simulink model "H2DFRL_LExCI_env_2018a"  (R2018a)
settings: Solver=FixedStepAuto  StartTime=0.0  StopTime=50  FixedStep=0.08  RelTol=1e-3
values from neighbouring files (symbols this model uses):
  action_mean_selector_ppo = 1:num_actions    [ReinforcementLearningBlockInit_H2DFRL.m]
  action_sampling_mode = 1    [ReinforcementLearningBlockInit_H2DFRL.m]
  action_selector_ddpg = 1:num_actions    [ReinforcementLearningBlockInit_H2DFRL.m]
  action_std_selector_ppo = 1:num_actions    [ReinforcementLearningBlockInit_H2DFRL.m]
  action_type = 1    [ReinforcementLearningBlockInit_H2DFRL.m]
  C2C_NMPC = init_C2C_NMPC_H2DF(C2C_NMPC.expdata)    [init_H2DFRL_GRU.m]
  num_actions = 4    [ReinforcementLearningBlockInit_H2DFRL.m]
  rl_algorithm = 1    [ReinforcementLearningBlockInit_H2DFRL.m]
undefined symbols (not defined in the file or in its folder): CA50_offset, DiscIntNeverNeededParam, enable_CA50_noise, enable_CA50_offset, enable_IMEP_noise, enable_IMEP_offset, IMEP_offset, NUMBER_OF_ACTIONS
libraries: simulink x15, dspsrcs4 x4
(part 2 of 3)

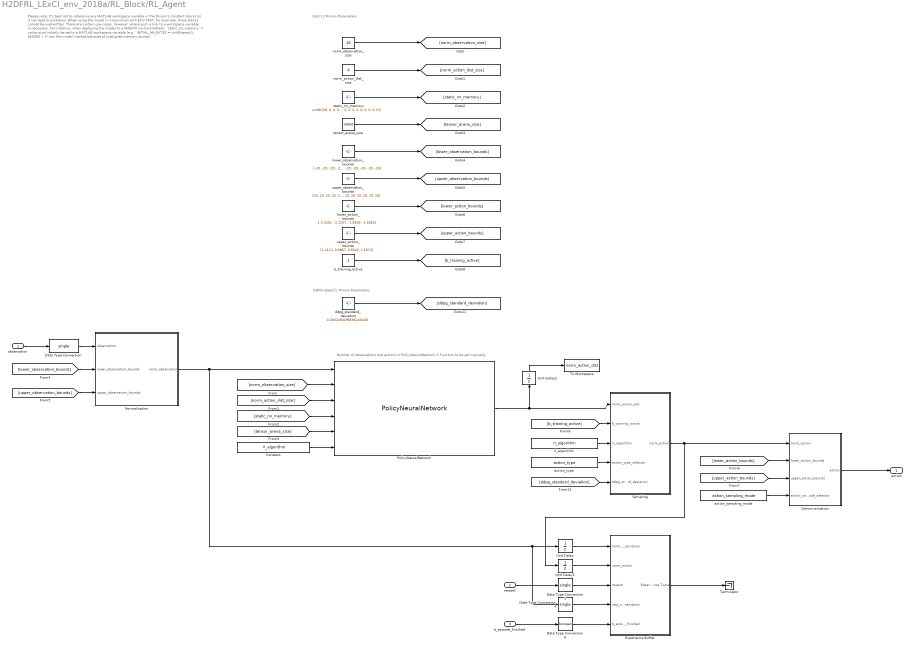
== system H2DFRL_LExCI_env_2018a/RL_Block/RL_Agent ==
  note: LExCI 2 Minion Parameters
  note: DDPG-Specific Minion Parameters
  note: Number of observations and actions in PolicyNeuralNetwork S-Function to be set manually.
  note: Please note:
      |
      | It's best not to reference any MATLAB workspace variable in the Minion's constant blocks as it can lead to
      | problems. When using the model in conjunction with ECU-TEST, for example, those blocks cannot be
      | overwritten.
      |
      | There are certain use-cases, however, where such a link to a workspace variable is necessary. For
      | instance, when deploying the model to a MABXIII via ControlDesk, `static_nn_memory`'s value must
      | initially be set to a MATLAB workspace variable (e.g. `INITIAL_NN_BYTES = uint8(zeros(1, 65536))`). If
      | not, the model crashes because of unaligned memory access.
  observation : Inport
  reward : Inport  Port=2
  b_episode_finished : Inport  Port=3
  Constant : Constant  Value=rl_algorithm  OutDataTypeStr=uint32
  Data Type Conversion : DataTypeConversion  OutDataTypeStr=single
  Data Type Conversion3 : DataTypeConversion  OutDataTypeStr=single
  Data Type Conversion4 : DataTypeConversion  OutDataTypeStr=single
  Data Type Conversion6 : DataTypeConversion  OutDataTypeStr=boolean
  Denormalization : Subsystem
  Experience Buffer : Subsystem
  Normalization : Subsystem
  PolicyNeuralNetwork : S-Function  InitFcn=try, set_param(gcb,'FunctionName','PolicyNeuralNetwork'), end  FunctionName=PolicyNeuralNetwork  SFunctionModules=PolicyNeuralNetwork_wrapper.cpp activations activations_common add add_common add_n arg_min_max assign_variable batch_to_space_nd broadcast_args broadcast_to call_once cast ceil circular_buffer circular_buffer_common comparisons concatenation conv conv_common cumsum depth_to_space depthwise_conv depthwise_conv_common dequantize dequantize_common detection_postprocess div elementwise elu ethosu exp expand_dims fill floor floor_div floor_mod fully_connected fully_connected_common gather gather_nd hard_swish hard_swish_common if kernel_runner kernel_util_micro l2norm l2_pool_2d leaky_relu leaky_relu_common logical logical_common logistic logistic_common log_softmax lstm_eval maximum_minimum micro_tensor_utils mirror_pad mul mul_common neg pack pad pooling pooling_common prelu prelu_common quantize quantize_common read_variable reduce reduce_common reshape resize_bilinear resize_nearest_neighbor round shape slice softmax softmax_common space_to_batch_nd space_to_depth split split_v squared_difference squeeze strided_slice sub sub_common svdf svdf_common tanh transpose transpose_conv unidirectional_sequence_lstm unpack var_handle while zeros_like flatbuffer_conversions op_resolver tensor_utils error_reporter schema_utils kernel_util portable_tensor_utils quantization_util common memory_helpers all_ops_resolver micro_graph micro_error_reporter micro_context micro_profiler test_helpers recording_micro_allocator micro_interpreter micro_time micro_resource_variable test_helper_custom_ops flatbuffer_utils mock_micro_graph debug_log micro_allocation_info system_setup micro_allocator micro_string micro_utils fake_micro_context persistent_arena_buffer_allocator recording_single_arena_buffer_allocator non_persistent_arena_buffer_allocator single_arena_buffer_allocator greedy_memory_planner linear_memory_planner non_persistent_buffer_planner_shim  SFunctionDeploymentMode=off  EnableBusSupport=off  mask(S-Function Builder){}
      mask help: Simulink:masks:SFunctionBuilder_MD
      mask init:
      | val = [[.9  0.75 0.75 1 1 .9 .9 1]',[1 1 0.75 0.75 .9 .9 1 .9]'];try , sys = get_param(gcb,'SfunBuilderFcnName');if isempty(sys), sys = get_param(gcb,'FunctionName'); end,catch, sys = get_param(gcb,'FunctionName'); end
      settings: CopyFcn=set_param(gcbh,'LinkStatus','none')  PreSaveFcn=try, set_param(gcb,'FunctionName','PolicyNeuralNetwork'), end  OpenFcn=sfunctionwizard(gcbh)
      mask Display: plot(val(:,1),val(:,2)),disp(sys),port_label('input',1,'norm_observation'),port_label('input',2,'norm_observation_size'),port_label('input',3,'norm_action_dist_size'),port_label('input',4,'static_nn_memory'),port_label('input',5,'tensor_arena_size'),port_label('input',6,'rl_algorithm'),port_label('output',1,'norm_action_dist')
  Sampling : Subsystem
  Terminator : Terminator
  To Workspace : ToWorkspace  VariableName=norm_action_dist  SampleTime=-1
  Unit Delay : UnitDelay  InitialCondition=-1*ones(16,1)  SampleTime=-1  HasFrameUpgradeWarning=on
  Unit Delay1 : UnitDelay  InitialCondition=-1*ones(4,1)  SampleTime=-1  HasFrameUpgradeWarning=on
  Unit Delay2 : UnitDelay  InitialCondition=-1*ones(4,1)  SampleTime=-1  HasFrameUpgradeWarning=on
  action_sampling_mode : Constant  Value=action_sampling_mode  OutDataTypeStr=uint8
  action_type : Constant  Value=action_type  OutDataTypeStr=uint8
  b_training_active : Constant  OutDataTypeStr=boolean
  ddpg_standard_deviation : Constant  Value=0.0002450298596240448  OutDataTypeStr=single
  lower_action_bounds : Constant  Value=[-2.3201, -2.1257, -1.8309, -1.6562]  OutDataTypeStr=single
  lower_observation_bounds : Constant  Value=[-20, -20, -20, -20, -20, -20, -20, -20, -20, -20, -20, -20, -20, -20, -20, -20]  OutDataTypeStr=single
  norm_action_dist_size : Constant  Value=4  OutDataTypeStr=uint32
  norm_observation_size : Constant  Value=16  OutDataTypeStr=uint32
  rl_algorithm : Constant  Value=rl_algorithm  OutDataTypeStr=uint8
  static_nn_memory : Constant  Value=uint8([28, 0, 0, 0, 84, 70, 76, 51, 0, 0, 18, 0, 28, 0, 24, 0, 20, 0, 16, 0, 12, 0, 8, 0, 0, 0, 4, 0, 18, 0, 0, 0, 24, 0, 0, 0, 104, 0, 0, 0, 140, 87, 0, 0, 156, 87, 0, 0, 228, 91, 0, 0, 3, 0, 0, 0, 2, 0, 0, 0, 44, 0, 0, 0, 4, 0, 0, 0, 40, 167, 255, 255, 12, 0, 0, 0, 4, 0, 0, 0, 19, 0, 0, 0, 67, 79, 78, 86, 69, 82, 83, 73, 79, 78, 95, 77, 69, 84, 65, 68, 65, 84, 65, 0, 76, 167, 255, 255, 11, 0, 0, 0, 4, 0, 0, 0, 19, 0, 0, 0, 109, 105, 110, 95, 114, 117, 110, 116, 105, 109, 101, 95, 118, 101, 114, 115, 105, 111, 110, 0, 13, 0, 0, 0, 32, 87, 0, 0, 0, 87, 0, 0, 232, 82, 0, 0, 216, 81, 0, 0, 200, 17, 0, 0, 184, 16, 0, 0, 168, 0, 0, 0, 160, 0, 0, 0, 152, 0, 0, 0, 144, 0, 0, 0, 136, 0, 0, 0, 104, 0, 0, 0, 4, 0, 0, 0, 54, 169, 255, 255, 4, 0, 0, 0, 84, 0, 0, 0, 12, 0, 0, 0, 8, 0, 14, 0, 8, 0, 4, 0, 8, 0, 0, 0, 16, 0, 0, 0, 36, 0, 0, 0, 0, 0, 6, 0, 8, 0, 4, 0, 6, 0, 0, 0, 4, 0, 0, 0, 0, 0, 0, 0, 0, 0, 10, 0, 16, 0, 12, 0, 8, 0, 4, 0, 10, 0, 0, 0, 2, 0, 0, 0, 2, 0, 0, 0, 4, 0, 0, 0, 6, 0, 0, 0, 50, 46, 49, 49, 46, 48, 0, 0, 150, 169, 255, 255, 4, 0, 0, 0, 16, 0, 0, 0, 49, 46, 53, 46, 48, 0, 0, 0, 0, 0, 0, 0, 0, 0, 0, 0, 80, 165, 255, 255, 84, 165, 255, 255, 88, 165, 255, 255, 92, 165, 255, 255, 194, 169, 255, 255, 4, 0, 0, 0, 0, 16, 0, 0, 195, 223, 248, 189, 165, 31, 134, 190, 238, 188, 71, 190, 121, 25, 100, 61, 240, 30, 182, 62, 66, 76, 196, 62, 202, 153, 72, 62, 139, 246, 211, 62, 185, 186, 23, 62, 196, 184, 59, 187, 236, 226, 53, 62, 128, 12, 9, 62, 67, 184, 120, 190, 173, 251, 162, 61, 146, 161, 55, 62, 148, 61, 179, 61, 220, 26, 78, 190, 129, 180, 236, 189, 201, 75, 95, 190, 158, 183, 249, 189, 54, 96, 9, 63, 14, 146, 237, 62, 146, 198, 19, 62, 129, 196, 40, 63, 237, 95, 204, 61, 193, 152, 236, 61, 42, 40, 87, 61, 27, 65, 222, 61, 75, 187, 23, 190, 145, 60, 6, 62, 176, 168, 115, 61, 9, 169, 14, 62, 178, 221, 16, 61, 40, 251, 84, 61, 173, 58, 218, 189, 173, 130, 55, 62, 66, 127, 175, 189, 163, 58, 143, 59, 62, 42, 119, 61, 238, 82, 2, 62, 197, 39, 121, 62, 149, 60, 136, 189, 43, 33, 133, 62, 37, 46, 138, 62, 207, 215, 141, 190, 123, 245, 155, 62, 8, 30, 68, 62, 158, 180, 235, 61, 208, 166, 161, 61, 149, 201, 38, 62, 58, 138, 138, 189, 132, 114, 22, 62, 87, 177, 14, 190, 95, 209, 112, 189, 153, 43, 92, 62, 219, 59, 206, 190, 251, 32, 146, 62, 215, 51, 11, 190, 77, 12, 196, 62, 154, 209, 132, 62, 62, 222, 11, 190, 169, 62, 196, 62, 85, 110, 63, 62, 70, 156, 153, 60, 0, 215, 9, 61, 240, 192, 152, 61, 101, 51, 8, 190, 245, 78, 254, 61, 14, 160, 180, 190, 189, 234, 120, 190, 128, 175, 63, 62, 207, 129, 172, 190, 72, 104, 114, 62, 219, 28, 40, 190, 84, 172, 109, 62, 27, 181, 89, 62, 231, 235, 87, 190, 181, 34, 153, 62, 147, 23, 127, 62, 157, 10, 130, 61, 147, 135, 36, 190, 239, 226, 30, 190, 80, 47, 40, 189, 86, 91, 51, 189, 110, 248, 200, 62, 7, 41, 241, 62, 235, 51, 3, 187, 10, 200, 189, 62, 218, 181, 5, 190, 101, 48, 201, 61, 160, 76, 118, 189, 176, 136, 228, 189, 9, 97, 195, 187, 34, 234, 10, 189, 82, 36, 249, 189, 145, 186, 35, 61, 188, 229, 86, 143, 182, 170, 85, 15, 145, 97, 86, 143, 66, 134, 85, 15, 254, 195, 85, 143, 65, 22, 87, 15, 151, 144, 87, 143, 177, 113, 87, 15, 93, 245, 86, 15, 209, 22, 86, 143, 135, 171, 85, 15, 121, 163, 85, 143, 135, 100, 86, 15, 52, 200, 86, 143, 40, 196, 85, 15, 231, 2, 86, 143, 222, 9, 169, 189, 75, 42, 168, 190, 121, 123, 65, 190, 4, 3, 14, 190, 237, 173, 137, 61, 132, 132, 136, 62, 147, 2, 62, 62, 92, 48, 196, 61, 212, 87, 131, 62, 170, 57, 42, 189, 236, 116, 7, 62, 253, 56, 164, 62, 194, 146, 151, 190, 98, 231, 50, 62, 26, 70, 103, 62, 112, 48, 97, 62, 230, 155, 179, 189, 198, 148, 87, 190, 118, 128, 40, 190, 203, 20, 148, 61, 72, 188, 226, 61, 38, 91, 27, 62, 49, 189, 5, 63, 230, 107, 37, 62, 146, 8, 130, 61, 173, 107, 137, 189, 148, 122, 55, 62, 186, 60, 98, 62, 160, 71, 42, 190, 76, 198, 104, 62, 241, 27, 26, 62, 172, 122, 0, 62, 153, 68, 86, 15, 232, 189, 85, 143, 124, 217, 85, 143, 252, 242, 85, 15, 17, 20, 86, 15, 29, 11, 87, 143, 243, 185, 85, 143, 5, 94, 86, 143, 226, 31, 86, 15, 230, 212, ...(+226621 chars)])  OutDataTypeStr=uint8
  tensor_arena_size : Constant  Value=100000  OutDataTypeStr=uint32
  upper_action_bounds : Constant  Value=[1.4113, 0.9867, 0.9542, 2.1874]  OutDataTypeStr=single
  upper_observation_bounds : Constant  Value=[20, 20, 20, 20, 20, 20, 20, 20, 20, 20, 20, 20, 20, 20, 20, 20]  OutDataTypeStr=single
  action : Outport
  wires:
  upper_action_bounds/1 -> [upper_action_bounds]
  PolicyNeuralNetwork/1 -> Unit Delay2/1, Sampling/1(norm_action_dist)
  upper_observation_bounds/1 -> [upper_observation_bounds]
  lower_action_bounds/1 -> [lower_action_bounds]
  [upper_observation_bounds] -> Normalization/3(upper_observation_bounds)
  [tensor_arena_size] -> PolicyNeuralNetwork/5
  b_episode_finished/1 -> Data Type Conversion6/1
  Unit Delay/1 -> Experience Buffer/1(norm_observation)
  [norm_observation_size] -> PolicyNeuralNetwork/2
  Data Type Conversion6/1 -> Experience Buffer/5(b_episode_finished)
  Unit Delay1/1 -> Experience Buffer/2(norm_action)
  Data Type Conversion3/1 -> Experience Buffer/3(reward)
  norm_observation_size/1 -> [norm_observation_size]
  Data Type Conversion/1 -> Normalization/1(observation)
  lower_observation_bounds/1 -> [lower_observation_bounds]
  Data Type Conversion4/1 -> Experience Buffer/4(new_norm_observation)
  reward/1 -> Data Type Conversion3/1
  norm_action_dist_size/1 -> [norm_action_dist_size]
  static_nn_memory/1 -> [static_nn_memory]
  Normalization/1(norm_observation) -> Unit Delay/1, Data Type Conversion4/1, PolicyNeuralNetwork/1
  observation/1 -> Data Type Conversion/1
  [norm_action_dist_size] -> PolicyNeuralNetwork/3
  [lower_observation_bounds] -> Normalization/2(lower_observation_bounds)
  tensor_arena_size/1 -> [tensor_arena_size]
  Experience Buffer/1(Experience Tuple) -> Terminator/1
  Sampling/1(norm_action) -> Unit Delay1/1, Denormalization/1(norm_action)
  Denormalization/1(action) -> action/1
  [lower_action_bounds] -> Denormalization/2(lower_action_bounds)
  [upper_action_bounds] -> Denormalization/3(upper_action_bounds)
  [static_nn_memory] -> PolicyNeuralNetwork/4
  b_training_active/1 -> [b_training_active]
  [b_training_active] -> Sampling/2(b_training_active)
  ddpg_standard_deviation/1 -> [ddpg_standard_deviation]
  action_sampling_mode/1 -> Denormalization/4(action_sampling_mode_selector)
  action_type/1 -> Sampling/4(action_type_selector)
  rl_algorithm/1 -> Sampling/3(rl_algorithm)
  [ddpg_standard_deviation] -> Sampling/5(ddpg_standard_deviation)
  Constant/1 -> PolicyNeuralNetwork/6
  Unit Delay2/1 -> To Workspace/1
